simulink model "counter_16ip_16ch"  (Simulink 6.2)
settings: Solver=ode45  StartTime=0.0  StopTime=20000  RelTol=1e-3
undefined symbols (not defined in the file or in its folder): iBOB
libraries: xbsIndex_r3 x119, xps_library x42, casper_library x13
(part 2 of 2)

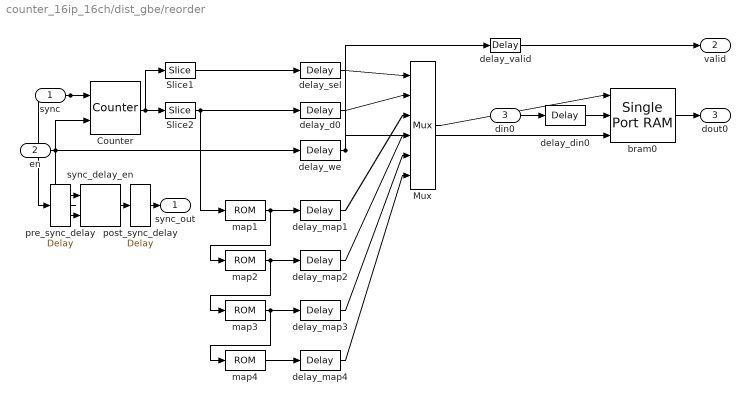
== system counter_16ip_16ch/dist_gbe/reorder ==
  sync : Inport  Port=1  LatchInput=off
  en : Inport  Port=2  LatchInput=off
  din0 : Inport  Port=3  LatchInput=off
  Counter : xbsIndex_r3/Counter  cnt_type=Count Limited  n_bits=13  bin_pt=0  arith_type=Unsigned  start_count=0  cnt_to=5119  cnt_by_val=1  operation=Up  explicit_period=off  period=1  load_pin=off  rst=on  en=on  dbl_ovrd=off  show_param=off  use_rpm=on  gen_core=off
      settings: xl_area=[0, 0, 0, 0, 0, 0, 0]
  Mux : xbsIndex_r3/Mux  inputs=5  precision=Full  arith_type="Signed  (2's comp)"  n_bits=8  bin_pt=2  quantization=Truncate  overflow=Wrap  latency=1  explicit_period=off  period=1  en=off  dbl_ovrd=off  show_param=off  mux_type=off  use_rpm=off  gen_core=off
      settings: xl_area=[0, 0, 0, 0, 0, 0, 0]
  Slice1 : xbsIndex_r3/Slice  mode=Upper Bit Location + Width  nbits=3  bit1=0  base1=MSB of Input  bit0=0  base0=LSB of Input  boolean_output=off  explicit_period=off  period=1  dbl_ovrd=off
  Slice2 : xbsIndex_r3/Slice  mode=Lower Bit Location + Width  nbits=10  bit1=0  base1=MSB of Input  bit0=0  base0=LSB of Input  boolean_output=off  explicit_period=off  period=1  dbl_ovrd=off
  bram0 : xbsIndex_r3/Single Port RAM  depth=1024  initVector=sin(pi*(0:15)/16)  write_mode=Read Before Write  latency=2  init_zero=on  explicit_period=off  period=1  rst=off  init_reg=0  en=off  dbl_ovrd=off  show_param=off  distributed_mem=off  use_rpm=off  gen_core=off
      settings: xl_area=[0, 0, 0, 0, 0, 0, 0]
  delay_d0 : xbsIndex_r3/Delay  latency=4  reg_retiming=off  explicit_period=off  period=1  en=off  accept_only_valid=off  init_zero=on  dbl_ovrd=off  show_param=off
      settings: xl_area=[0, 0, 0, 0, 0, 0, 0]
  delay_din0 : xbsIndex_r3/Delay  latency=5  reg_retiming=off  explicit_period=off  period=1  en=off  accept_only_valid=off  init_zero=on  dbl_ovrd=off  show_param=off
      settings: xl_area=[0, 0, 0, 0, 0, 0, 0]
  delay_map1 : xbsIndex_r3/Delay  latency=3*map_latency  reg_retiming=off  explicit_period=off  period=1  en=off  accept_only_valid=off  init_zero=on  dbl_ovrd=off  show_param=off
      settings: xl_area=[0, 0, 0, 0, 0, 0, 0]
  delay_map2 : xbsIndex_r3/Delay  latency=2*map_latency  reg_retiming=off  explicit_period=off  period=1  en=off  accept_only_valid=off  init_zero=on  dbl_ovrd=off  show_param=off
      settings: xl_area=[0, 0, 0, 0, 0, 0, 0]
  delay_map3 : xbsIndex_r3/Delay  latency=1*map_latency  reg_retiming=off  explicit_period=off  period=1  en=off  accept_only_valid=off  init_zero=on  dbl_ovrd=off  show_param=off
      settings: xl_area=[0, 0, 0, 0, 0, 0, 0]
  delay_map4 : xbsIndex_r3/Delay  latency=0*map_latency  reg_retiming=off  explicit_period=off  period=1  en=off  accept_only_valid=off  init_zero=on  dbl_ovrd=off  show_param=off
      settings: xl_area=[0, 0, 0, 0, 0, 0, 0]
  delay_sel : xbsIndex_r3/Delay  latency=4  reg_retiming=off  explicit_period=off  period=1  en=off  accept_only_valid=off  init_zero=on  dbl_ovrd=off  show_param=off
      settings: xl_area=[0, 0, 0, 0, 0, 0, 0]
  delay_valid : xbsIndex_r3/Delay  latency=3  reg_retiming=off  explicit_period=off  period=1  en=off  accept_only_valid=off  init_zero=on  dbl_ovrd=off  show_param=off
      settings: xl_area=[0, 0, 0, 0, 0, 0, 0]
  delay_we : xbsIndex_r3/Delay  latency=4  reg_retiming=off  explicit_period=off  period=1  en=off  accept_only_valid=off  init_zero=on  dbl_ovrd=off  show_param=off
      settings: xl_area=[0, 0, 0, 0, 0, 0, 0]
  map{1..4} (4 alike) : xbsIndex_r3/ROM  depth=1024  initVector=[0 16 32 48 64 80 96 112 128 144 160 176 192 208 224 240 256 272 288 304 320 336 352 368 384 400 416 432 448 464 480 496 512 528 544 560 576 592 608 624 640 656 672 688 704 720 736 752 768 784 800 816 832 848 864 880 896 912 928 944 960 976 992 1008 1 17 33 49 65 81 97 113 129 145 161 177 193 209 225 241 257 273 289 305 321 337 353 369 385 401 417 433 449 465 481 497 513 529 545 561 577 593 609 625 641 657 673 689 705 721 737 753 769 785 801 817 833 849 865 881 897 913 929 945 961 977 993 1009 2 18 34 50 66 82 98 114 130 146 162 178 194 210 226 242 258 274 290 306 322 338 354 370 386 402 418 434 450 466 482 498 514 530 546 562 578 594 610 626 642 658 674 690 706 722 738 754 770 786 802 818 834 850 866 882 898 914 930 946 962 978 994 1010 3 19 35 51 67 83 99 115 131 147 163 179 195 211 227 243 259 275 291 307 323 339 355 371 387 403 419 435 451 467 483 499 515 531 547 563 579 595 611 627 643 659 675 691 707 723 739 755 771 787 803 819 835 851 867 883 899 915 931 947 963 979 995 1011 4 20 36 52 68 84 100 116 132 148 164 180 196 212 228 244 260 276 292 308 324 340 356 372 388 404 420 436 452 468 484 500 516 532 548 564 580 596 612 628 644 660 676 692 708 724 740 756 772 788 804 820 836 852 868 884 900 916 932 948 964 980 996 1012 5 21 37 53 69 85 101 117 133 149 165 181 197 213 229 245 261 277 293 309 325 341 357 373 389 405 421 437 453 469 485 501 517 533 549 565 581 597 613 629 645 661 677 693 709 725 741 757 773 789 805 821 837 853 869 885 901 917 933 949 965 981 997 1013 6 22 38 54 70 86 102 118 134 150 166 182 198 214 230 246 262 278 294 310 326 342 358 374 390 406 422 438 454 470 486 502 518 534 550 566 582 598 614 630 646 662 678 694 710 726 742 758 774 790 806 822 838 854 870 886 902 918 934 950 966 982 998 1014 7 23 39 55 71 87 103 119 135 151 167 183 199 215 231 247 263 279 295 311 327 343 359 375 391 407 423 439 455 471 487 503 519 535 551 567 583 599 615 631 647 663 679 695 711 727 743 759 775 791 807 823 839 855 871 887 903 919 935 951 967 983 999 1015 8 24 40 56 72 88 104 120 136 152 168 184 200 216 232 248 264 280 296 312 328 344 360 376 392 408 424 440 456 472 488 504 520 536 552 568 584 600 616 632 648 664 680 696 712 728 744 760 776 792 808 824 840 856 872 888 904 920 936 952 968 984 1000 1016 9 25 41 57 73 89 105 121 137 153 169 185 201 217 233 249 265 281 297 313 329 345 361 377 393 409 425 441 457 473 489 505 521 537 553 569 585 601 617 633 649 665 681 697 713 729 745 761 777 793 809 825 841 857 873 889 905 921 937 953 969 985 1001 1017 10 26 42 58 74 90 106 122 138 154 170 186 202 218 234 250 266 282 298 314 330 346 362 378 394 410 426 442 458 474 490 506 522 538 554 570 586 602 618 634 650 666 682 698 714 730 746 762 778 794 810 826 842 858 874 890 906 922 938 954 970 986 1002 1018 11 27 43 59 75 91 107 123 139 155 171 187 203 219 235 251 267 283 299 315 331 347 363 379 395 411 427 443 459 475 491 507 523 539 555 571 587 603 619 635 651 667 683 699 715 731 747 763 779 795 811 827 843 859 875 891 907 923 939 955 971 987 1003 1019 12 28 44 60 76 92 108 124 140 156 172 188 204 220 236 252 268 284 300 316 332 348 364 380 396 412 428 444 460 476 492 508 524 540 556 572 588 604 620 636 652 668 684 700 716 732 748 764 780 796 812 828 844 860 876 892 908 924 940 956 972 988 1004 1020 13 29 45 61 77 93 109 125 141 157 173 189 205 221 237 253 269 285 301 317 333 349 365 381 397 413 429 445 461 477 493 509 525 541 557 573 589 605 621 637 653 669 685 701 717 733 749 765 781 797 813 829 845 861 877 893 909 925 941 957 973 989 1005 1021 14 30 46 62 78 94 110 126 142 158 174 190 206 222 238 254 270 286 302 318 334 350 366 382 398 414 430 446 462 478 494 510 526 542 558 574 590 606 622 638 654 670 686 702 718 734 750 766 782 798 814 830 846 862 878 894 910 926 942 958 974 990 1006 1022 15 31 47 63 79 95 111 127 143 159 175 191 207 223 239 255 271 287 303 319 335 351 367 383 399 415 431 447 463 479 495 511 527 543 559 575 591 607 623 639 655 671 687 703 719 735 751 767 783 799 815 831 847 863 879 895 911 927 943 959 975 991 1007 1023]  arith_type=Unsigned  n_bits=10  bin_pt=0  latency=1  init_zero=on  explicit_period=off  period=1  rst=off  init_reg=0  en=off  dbl_ovrd=off  show_param=off  distributed_mem=on  use_rpm=off  gen_core=off
      settings: xl_area=[0, 0, 0, 0, 0, 0, 0]
  post_sync_delay : xbsIndex_r3/Delay  latency=3  reg_retiming=off  explicit_period=off  period=1  en=off  accept_only_valid=off  init_zero=on  dbl_ovrd=off  show_param=off
      settings: xl_area=[0, 0, 0, 0, 0, 0, 0]
  pre_sync_delay : xbsIndex_r3/Delay  latency=4  reg_retiming=off  explicit_period=off  period=1  en=off  accept_only_valid=off  init_zero=on  dbl_ovrd=off  show_param=off
      settings: xl_area=[0, 0, 0, 0, 0, 0, 0]
  sync_delay_en : casper_library/Delays/sync_delay_en  DelayLen=1024
      link override Constant: equ=P=C
      link override Constant1: equ=P=C
      link override Constant2: equ=P=C
      link override Constant3: equ=P=C
  sync_out : Outport
  valid : Outport  Port=2
  dout0 : Outport  Port=3
  wires:
  sync/1 -> Counter/1, pre_sync_delay/1
  en/1 -> Counter/2, sync_delay_en/2, delay_we/1
  Counter/1 -> Slice1/1, Slice2/1
  Slice1/1 -> delay_sel/1
  delay_sel/1 -> Mux/1
  Slice2/1 -> delay_d0/1, map1/1
  delay_d0/1 -> Mux/2
  pre_sync_delay/1 -> sync_delay_en/1
  sync_delay_en/1 -> post_sync_delay/1
  post_sync_delay/1 -> sync_out/1
  delay_we/1 -> delay_valid/1, bram0/3
  delay_valid/1 -> valid/1
  Mux/1 -> bram0/1
  din0/1 -> delay_din0/1
  delay_din0/1 -> bram0/2
  bram0/1 -> dout0/1
  map1/1 -> delay_map1/1, map2/1
  delay_map1/1 -> Mux/3
  map2/1 -> delay_map2/1, map3/1
  delay_map2/1 -> Mux/4
  map3/1 -> delay_map3/1, map4/1
  delay_map3/1 -> Mux/5
  map4/1 -> delay_map4/1
  delay_map4/1 -> Mux/6
